simulink model "FWT_Plant"  (R2020b)
settings: Solver=ode45  StartTime=0.0  StopTime=600  MaxStep=12.0  RelTol=1e-3
values from neighbouring files (symbols this model uses):
  g13 = tf(num(1,:),den)    [RCA2.m]
  Gdss = ss(Gd)    [RCA2.m]
  Gss = ss(A2,B2,C2,D2)    [RCA2.m]
  K2ss = minreal(K2ss)    [RCA2.m]
  Kdss = minreal(Kdss)    [RCA2.m]
  W = minreal(ss([g13;g23]))    [RCA2.m]
settings Model: Creator=Work  LastModifiedBy=Work

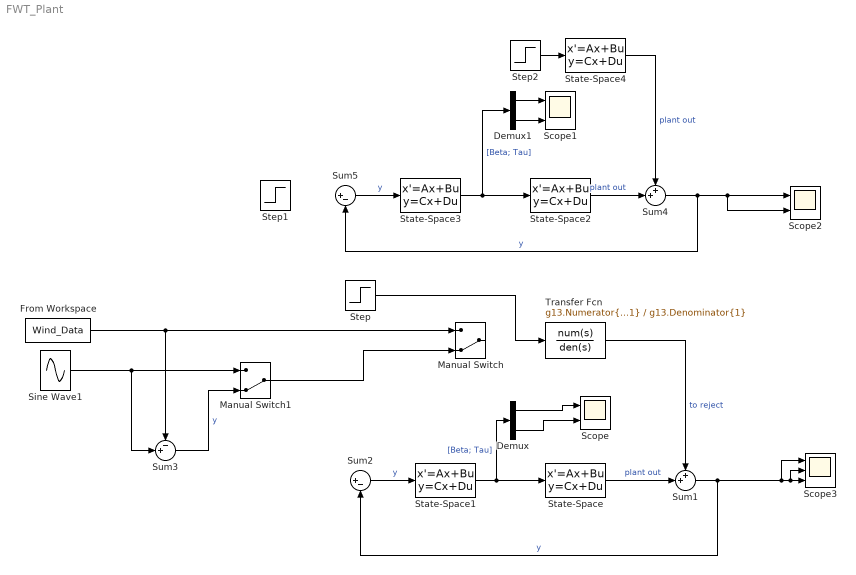
== system FWT_Plant ==
  Demux : Demux  Outputs=2
  Demux1 : Demux  Outputs=2
  From Workspace : FromWorkspace  VariableName=Wind_Data
  Manual Switch : ManualSwitch  CurrentSetting=0
  Manual Switch1 : ManualSwitch  CurrentSetting=0
  Scope : Scope  NumInputPorts=2
  Scope1 : Scope  NumInputPorts=2
  Scope2 : Scope  NumInputPorts=2
  Scope3 : Scope  NumInputPorts=3
  Sine Wave1 : Sin  Amplitude=2  Frequency=0.00628  SampleTime=0
  State-Space : StateSpace  A=Gdss.A  B=Gdss.B  C=Gdss.C  D=Gdss.D  InitialCondition=0
  State-Space1 : StateSpace  A=Kdss.A  B=Kdss.B  C=Kdss.C  D=Kdss.D  InitialCondition=0
  State-Space2 : StateSpace  A=Gss.A  B=Gss.B  C=Gss.C  D=Gss.D  InitialCondition=0
  State-Space3 : StateSpace  A=K2ss.A  B=K2ss.B  C=K2ss.C  D=K2ss.D  InitialCondition=0
  State-Space4 : StateSpace  A=W.A  B=W.B  C=W.C  D=W.D  InitialCondition=0
  Step : Step  Time=100  SampleTime=0
  Step1 : Step  Time=100  SampleTime=0
  Step2 : Step  Time=100  SampleTime=0
  Sum1 : Sum  Inputs=++|
  Sum2 : Sum  Inputs=|+-
  Sum3 : Sum  Inputs=-+|
  Sum4 : Sum  Inputs=++|
  Sum5 : Sum  Inputs=|+-
  Transfer Fcn : TransferFcn  Numerator=g13.Numerator{1}  Denominator=g13.Denominator{1}
  wires:
  State-Space/1 -> Sum1/2  "plant out"
  Sum1/1 -> Sum2/2, Scope3/1, Scope3/2, Scope3/3  "y"
  Sum2/1 -> State-Space1/1  "y"
  State-Space1/1 -> Demux/1, State-Space/1  "[Beta; Tau]"
  From Workspace/1 -> Manual Switch/1, Sum3/1
  Sine Wave1/1 -> Manual Switch1/1, Sum3/2
  Sum3/1 -> Manual Switch1/2  "y"
  Manual Switch1/1 -> Manual Switch/2
  Demux/2 -> Scope/2
  Demux/1 -> Scope/1
  Sum5/1 -> State-Space3/1  "y"
  State-Space3/1 -> State-Space2/1, Demux1/1  "[Beta; Tau]"
  Demux1/2 -> Scope1/2
  Demux1/1 -> Scope1/1
  State-Space2/1 -> Sum4/2  "plant out"
  Sum4/1 -> Sum5/2, Scope2/2, Scope2/1  "y"
  Step2/1 -> State-Space4/1
  State-Space4/1 -> Sum4/1  "plant out"
  Step/1 -> Transfer Fcn/1
  Transfer Fcn/1 -> Sum1/1  "to reject"
